simulink model "TBRe18_ECU_V6"  (R2015b)
settings: Solver=FixedStepDiscrete  SolverMode=SingleTasking  StartTime=0.0  StopTime=inf  FixedStep=0.0001  RelTol=1e-3
PostLoadFcn:
  | model_init();
libraries: simulink x20, simulink_extras x1
(part 2 of 4)

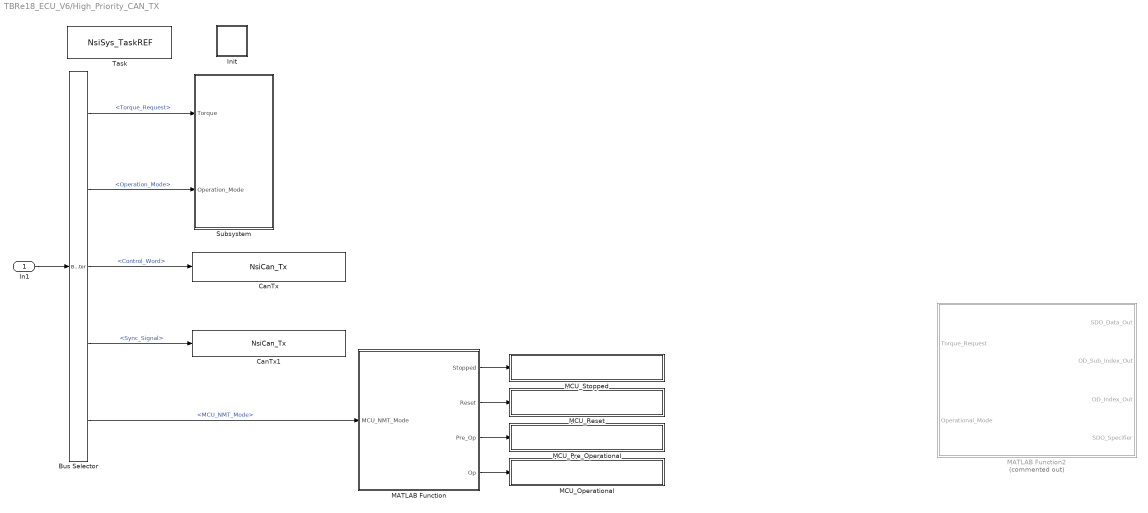
== system TBRe18_ECU_V6/High_Priority_CAN_TX ==
  In1 : Inport
  Bus Selector : BusSelector  OutputSignals=Drive_Data.Torque_Request,Vehicle_Operation_Data.Operation_Mode,Drive_Data.Control_Word,Drive_Data.Sync_Signal,Vehicle_Operation_Data.MCU_NMT_Mode
  CanTx : S-Function  FunctionName=NsiCan_Tx  Parameters=data_can,channel,msg_name,ident,ident_type,dlc,signals  SFunctionDeploymentMode=off  EnableBusSupport=off  mask(MUXlink Can Tx){data_can=1;HIGH_SPEED;500Kbps;120 Ohm;C:\Users\William\Documents\ECU\DBC\TBRe18_DBC_V1.dbc;0;1;HIGH_SPEED;500Kbps;120 Ohm;C:\Users\William\Documents\ECU\DBC\TBRe18_DBC_V1.dbc;0;0;HIGH_SPEED;500Kbps;120 Ohm;C:\Users\l\Desktop\FYP\ECU\DBC\TBRe_DBC_V2.dbc;0;0;HIGH_SPEED;500Kbps;120 Ohm;D:\TOOLS\MUXLINK\R2011b\MUXlink\misc\j1939_adapt.dbc;0;0;HIGH_SPEED;1000Kbps;No;D:\TOOLS\MUXLINK\R2011b\MUXlink\misc\BASE_CAN_MUXLAB4.dbc;0, channel=1, msg_name=MCU_RPDO1, ident=0x201, ident_type=STD, dlc=8, signals=MCU_ControlWord;1;0;16}
      mask prompts: data_can "data can"; msg_name "msg name"
      mask help: Transmit a frame on a CAN Channel.
      mask init:
      | NsiCan_Tx_InitializationFcn();
      settings: OpenFcn=NsiCan_Tx_OpenFcn();
      mask Help:
      | eval('block=get_param(gcb, ''RTWdata'');')
      | web([docroot '\toolbox\MUXlink\html\blocks/' block.MUXlink_BlockType '.html'])
      mask Callback data_can: NsiCan_Tx_ApplyFcn(1);
      mask Callback channel: NsiCan_Tx_ApplyFcn(2);
      mask Callback msg_name: NsiCan_Tx_ApplyFcn(3);
      mask Callback ident: NsiCan_Tx_ApplyFcn(4);
      mask Callback ident_type: NsiCan_Tx_ApplyFcn(5);
      mask Callback dlc: NsiCan_Tx_ApplyFcn(6);
      mask Callback signals: NsiCan_Tx_ApplyFcn(7);
      mask Display: image(imread('nsi.bmp'));text(0.5, 0.1, 'TX_MCU_RPDO1_CAN1', 'horizontalAlignment', 'center', 'verticalAlignment', 'base');plot([0.05 0.05 0.05 0.05 0.05 0.05 0.05 0.05 0.05 0.05]); port_label('input',1, 'MCU_ControlWord');
  CanTx1 : S-Function  FunctionName=NsiCan_Tx  Parameters=data_can,channel,msg_name,ident,ident_type,dlc,signals  SFunctionDeploymentMode=off  EnableBusSupport=off  mask(MUXlink Can Tx){data_can=1;HIGH_SPEED;500Kbps;120 Ohm;C:\Users\William\Documents\ECU\DBC\TBRe18_DBC_V1.dbc;0;1;HIGH_SPEED;500Kbps;120 Ohm;C:\Users\William\Documents\ECU\DBC\TBRe18_DBC_V1.dbc;0;0;HIGH_SPEED;500Kbps;120 Ohm;C:\Users\l\Desktop\FYP\ECU\DBC\TBRe_DBC_V2.dbc;0;0;HIGH_SPEED;500Kbps;120 Ohm;D:\TOOLS\MUXLINK\R2011b\MUXlink\misc\j1939_adapt.dbc;0;0;HIGH_SPEED;1000Kbps;No;D:\TOOLS\MUXLINK\R2011b\MUXlink\misc\BASE_CAN_MUXLAB4.dbc;0, channel=1, msg_name=MCU_Sync_MSG, ident=0x080, ident_type=STD, dlc=1, signals=Sync_Command;1;0;8}
      mask prompts: data_can "data can"; msg_name "msg name"
      mask help: Transmit a frame on a CAN Channel.
      mask init:
      | NsiCan_Tx_InitializationFcn();
      settings: OpenFcn=NsiCan_Tx_OpenFcn();
      mask Help:
      | eval('block=get_param(gcb, ''RTWdata'');')
      | web([docroot '\toolbox\MUXlink\html\blocks/' block.MUXlink_BlockType '.html'])
      mask Callback data_can: NsiCan_Tx_ApplyFcn(1);
      mask Callback channel: NsiCan_Tx_ApplyFcn(2);
      mask Callback msg_name: NsiCan_Tx_ApplyFcn(3);
      mask Callback ident: NsiCan_Tx_ApplyFcn(4);
      mask Callback ident_type: NsiCan_Tx_ApplyFcn(5);
      mask Callback dlc: NsiCan_Tx_ApplyFcn(6);
      mask Callback signals: NsiCan_Tx_ApplyFcn(7);
      mask Display: image(imread('nsi.bmp'));text(0.5, 0.1, 'TX_MCU_Sync_MSG_CAN1', 'horizontalAlignment', 'center', 'verticalAlignment', 'base');plot([0.05 0.05 0.05 0.05 0.05 0.05 0.05 0.05 0.05 0.05]); port_label('input',1, 'Sync_Command');
  Init : Subsystem  mask(System Initialize){}
      mask help: Add code to a systems Initialize function
      settings: CopyFcn=cccopyfcn(gcb)  OpenFcn=ccopenfcn('System Initialize Function')
      mask Help: This block contains text fields to insert custom user code sections at the declaration, execution and exit sections of the systems initialize function.  By placing this block inside a subsytem, the custom user code will appear in that subsystems function.
      mask Display: disp('I()')
  MATLAB Function : MATLAB Function  TreatAsAtomicUnit=on
  MATLAB Function2 : MATLAB Function  Commented=on  TreatAsAtomicUnit=on
  MCU_Operational : Subsystem
  MCU_Pre_Operational : Subsystem
  MCU_Reset : Subsystem
  MCU_Stopped : Subsystem
  Subsystem : Subsystem
  Task : S-Function  FunctionName=NsiSys_TaskREF  Parameters=task_initialised,task_periodic, task_sampletime,task_name,task_event,task_offset  SFunctionDeploymentMode=off  EnableBusSupport=off  mask(task definition){task_initialised=on, task_periodic=on, task_sampletime=[0.1], task_offset=0.03, task_name=High_Priority_CAN_TX, task_event=on}
      mask prompts: task_initialised "task initialised"; task_periodic "Is Periodic"; task_sampletime "Task sample time"; task_offset "Task Offset"; task_name "Task name"; task_event "Is event"
      mask help:
      | Permit to provide all parameters associated to a MUXLINK task.
      | Task can be executed periodicaly and/or on event detection.
      | If task is periodic:
      | Task sample time specify the execution period in mS [0.001   6000]
      | Task Offset specify the offset applied to the execution period
      | Task Offset < Task sample time
      mask init:
      | NsiSys_TaskREF_InitializationFcn();
      settings: OpenFcn=NsiSys_Task_OpenFcn();
      mask Callback task_initialised: NsiSys_TaskREF_ApplyFcn(1);
      mask Callback task_periodic: NsiSys_TaskREF_ApplyFcn(2);
      mask Callback task_sampletime: NsiSys_TaskREF_ApplyFcn(3);
      mask Callback task_offset: NsiSys_TaskREF_ApplyFcn(6);
      mask Callback task_name: NsiSys_TaskREF_ApplyFcn(4);
      mask Callback task_event: NsiSys_TaskREF_ApplyFcn(5);
      mask Display: text(0.5, 0.8, 't()', 'horizontalAlignment', 'center', 'verticalAlignment', 'base');text(0.5, 0.2, '/ 100.0ms / 30.0ms /', 'horizontalAlignment', 'center', 'verticalAlignment', 'base');text(0.5, 0.4, 'Event', 'horizontalAlignment', 'center', 'verticalAlignment', 'base');
  wires:
  In1/1 -> Bus Selector/1
  Bus Selector/4 -> CanTx1/1  "<Sync_Signal>"
  MATLAB Function/4(Op) -> MCU_Operational/Trigger
  MATLAB Function/1(Stopped) -> MCU_Stopped/Trigger
  MATLAB Function/3(Pre_Op) -> MCU_Pre_Operational/Trigger
  Bus Selector/5 -> MATLAB Function/1(MCU_NMT_Mode)  "<MCU_NMT_Mode>"
  Bus Selector/3 -> CanTx/1  "<Control_Word>"
  MATLAB Function/2(Reset) -> MCU_Reset/Trigger
  Bus Selector/2 -> Subsystem/2(Operation_Mode)  "<Operation_Mode>"
  Bus Selector/1 -> Subsystem/1(Torque)  "<Torque_Request>"

== system TBRe18_ECU_V6/Low_Priority_CAN_RX ==
  Bus Creator : BusCreator  Inputs=15
  Bus Creator1 : BusCreator  Inputs=11
  Bus Creator2 : BusCreator  Inputs=2
  CanRx : S-Function  FunctionName=NsiCan_Rx  Parameters=data_can,channel,msg_name,ident,ident_type,dlc,signals,is_trigger  SFunctionDeploymentMode=off  EnableBusSupport=off  mask(MUXlink Can Rx){data_can=1;HIGH_SPEED;500Kbps;120 Ohm;C:\Users\William\Documents\ECU\DBC\TBRe18_DBC_V1.dbc;0;;1;HIGH_SPEED;500Kbps;120 Ohm;C:\Users\William\Documents\ECU\DBC\TBRe18_DBC_V1.dbc;0;;0;HIGH_SPEED;500Kbps;120 Ohm;C:\Users\l\Desktop\FYP\ECU\DBC\TBRe_DBC_V2.dbc;0;;0;HIGH_SPEED;500Kbps;120 Ohm;D:\TOOLS\MUXLINK\R2011b\MUXlink\misc\j1939_adapt.dbc;0;;0;HIGH_SPEED;1000Kbps;No;D:\TOOLS\MUXLINK\R2011b\MUXlink\misc\BASE_CAN_MUXLAB4.dbc;0;, channel=2, msg_name=Shutdown_TPDO, ident=0x185, ident_type=STD, dlc=2, signals=High_AIR_Fault;1;13;1;TSMS_Fault;1;12;1;HVD_Fault;1;11;1;Front_Return_Fault;1;10;1;E2_Switch_Fault;1;9;1;E1_Switch_Fault;1;8;1;Latch_Out_Fault;1;7;1;Latch_In_Fault;1;6;1;BSPD_TSI_Fault;1;5;1;BSPD_Fault;1;4;1;IMD_Fault;1;3;1;BMS_Fault;1;2;1;ESTP_Right_Fault;1;1;1;ESTP_Left_Fault;1;0;1, is_trigger=0}
      mask prompts: data_can "data can"; msg_name "msg name"
      mask help: Receive a frame from a CAN channel.
      mask init:
      | NsiCan_Rx_InitializationFcn();
      settings: OpenFcn=NsiCan_Rx_OpenFcn();
      mask Help:
      | eval('block=get_param(gcb, ''RTWdata'');')
      | web([docroot '\toolbox\MUXlink\html\blocks/' block.MUXlink_BlockType '.html'])
      mask Callback data_can: NsiCan_Rx_ApplyFcn(1);
      mask Callback channel: NsiCan_Rx_ApplyFcn(2);
      mask Callback msg_name: NsiCan_Rx_ApplyFcn(3);
      mask Callback ident: NsiCan_Rx_ApplyFcn(4);
      mask Callback ident_type: NsiCan_Rx_ApplyFcn(5);
      mask Callback dlc: NsiCan_Rx_ApplyFcn(6);
      mask Callback signals: NsiCan_Rx_ApplyFcn(7);
      mask Callback is_trigger: NsiCan_Rx_ApplyFcn(8);
      mask Display: image(imread('nsi.bmp'));text(0.5, 0.3, 'RX_Shutdown_TPDO_CAN2', 'horizontalAlignment', 'center', 'verticalAlignment', 'base');plot([0.05 0.05 0.05 0.05 0.05 0.05 0.05 0.05 0.05 0.05]); port_label('output',1, 'High_AIR_Fault'); port_label('output',2, 'TSMS_Fault'); port_label('output',3, 'HVD_Fault'); port_label('output',4, 'Front_Return_Fault'); port_label('output',5, 'E2_Switch_Fault'); port_label('output',6, 'E1_Switch_Fault'); port_label('output',7, 'Latch_Out_Fault'); port_label('output',8, 'Latch_In_Fault'); port_label('output',9, 'BSPD_TSI_Fault'); port_label('output',10, 'BSPD_Fault'); port_label('output',11, 'IMD_Fault'); port_label('output',12, 'BMS_Fault'); port_label('output',13, 'ESTP_Right_Fault'); port_label('output',14, 'ESTP_Left_Fault'); port_label('output',15, 'Status');
  CanRx1 : S-Function  FunctionName=NsiCan_Rx  Parameters=data_can,channel,msg_name,ident,ident_type,dlc,signals,is_trigger  SFunctionDeploymentMode=off  EnableBusSupport=off  mask(MUXlink Can Rx){data_can=1;HIGH_SPEED;500Kbps;120 Ohm;C:\Users\William\Documents\ECU\DBC\TBRe18_DBC_V1.dbc;0;;1;HIGH_SPEED;500Kbps;120 Ohm;C:\Users\William\Documents\ECU\DBC\TBRe18_DBC_V1.dbc;0;;0;HIGH_SPEED;500Kbps;120 Ohm;C:\Users\l\Desktop\FYP\ECU\DBC\TBRe_DBC_V2.dbc;0;;0;HIGH_SPEED;500Kbps;120 Ohm;D:\TOOLS\MUXLINK\R2011b\MUXlink\misc\j1939_adapt.dbc;0;;0;HIGH_SPEED;1000Kbps;No;D:\TOOLS\MUXLINK\R2011b\MUXlink\misc\BASE_CAN_MUXLAB4.dbc;0;, channel=2, msg_name=BMS_Feedback_1, ident=0x050, ident_type=STD, dlc=7, signals=Instant_Pack_Voltage;1;0;16;Pack_SOC;1;16;16;Pack_Current;1;32;16;Acc_Fan_Speed;1;48;8, is_trigger=0}
      mask prompts: data_can "data can"; msg_name "msg name"
      mask help: Receive a frame from a CAN channel.
      mask init:
      | NsiCan_Rx_InitializationFcn();
      settings: OpenFcn=NsiCan_Rx_OpenFcn();
      mask Help:
      | eval('block=get_param(gcb, ''RTWdata'');')
      | web([docroot '\toolbox\MUXlink\html\blocks/' block.MUXlink_BlockType '.html'])
      mask Callback data_can: NsiCan_Rx_ApplyFcn(1);
      mask Callback channel: NsiCan_Rx_ApplyFcn(2);
      mask Callback msg_name: NsiCan_Rx_ApplyFcn(3);
      mask Callback ident: NsiCan_Rx_ApplyFcn(4);
      mask Callback ident_type: NsiCan_Rx_ApplyFcn(5);
      mask Callback dlc: NsiCan_Rx_ApplyFcn(6);
      mask Callback signals: NsiCan_Rx_ApplyFcn(7);
      mask Callback is_trigger: NsiCan_Rx_ApplyFcn(8);
      mask Display: image(imread('nsi.bmp'));text(0.5, 0.3, 'RX_BMS_Feedback_1_CAN2', 'horizontalAlignment', 'center', 'verticalAlignment', 'base');plot([0.05 0.05 0.05 0.05 0.05 0.05 0.05 0.05 0.05 0.05]); port_label('output',1, 'Instant_Pack_Voltage'); port_label('output',2, 'Pack_SOC'); port_label('output',3, 'Pack_Current'); port_label('output',4, 'Acc_Fan_Speed'); port_label('output',5, 'Status');
  CanRx2 : S-Function  FunctionName=NsiCan_Rx  Parameters=data_can,channel,msg_name,ident,ident_type,dlc,signals,is_trigger  SFunctionDeploymentMode=off  EnableBusSupport=off  mask(MUXlink Can Rx){data_can=1;HIGH_SPEED;500Kbps;120 Ohm;C:\Users\William\Documents\ECU\DBC\TBRe18_DBC_V1.dbc;0;;1;HIGH_SPEED;500Kbps;120 Ohm;C:\Users\William\Documents\ECU\DBC\TBRe18_DBC_V1.dbc;0;;0;HIGH_SPEED;500Kbps;120 Ohm;C:\Users\l\Desktop\FYP\ECU\DBC\TBRe_DBC_V2.dbc;0;;0;HIGH_SPEED;500Kbps;120 Ohm;D:\TOOLS\MUXLINK\R2011b\MUXlink\misc\j1939_adapt.dbc;0;;0;HIGH_SPEED;1000Kbps;No;D:\TOOLS\MUXLINK\R2011b\MUXlink\misc\BASE_CAN_MUXLAB4.dbc;0;, channel=2, msg_name=BMS_Feedback_2, ident=0x051, ident_type=STD, dlc=8, signals=Avg_Cell_Voltage;1;32;16;High_Cell_Voltage;1;16;16;High_Cell_ID;1;56;8;Low_Cell_Voltage;1;0;16;Low_Cell_ID;1;48;8, is_trigger=0}
      mask prompts: data_can "data can"; msg_name "msg name"
      mask help: Receive a frame from a CAN channel.
      mask init:
      | NsiCan_Rx_InitializationFcn();
      settings: OpenFcn=NsiCan_Rx_OpenFcn();
      mask Help:
      | eval('block=get_param(gcb, ''RTWdata'');')
      | web([docroot '\toolbox\MUXlink\html\blocks/' block.MUXlink_BlockType '.html'])
      mask Callback data_can: NsiCan_Rx_ApplyFcn(1);
      mask Callback channel: NsiCan_Rx_ApplyFcn(2);
      mask Callback msg_name: NsiCan_Rx_ApplyFcn(3);
      mask Callback ident: NsiCan_Rx_ApplyFcn(4);
      mask Callback ident_type: NsiCan_Rx_ApplyFcn(5);
      mask Callback dlc: NsiCan_Rx_ApplyFcn(6);
      mask Callback signals: NsiCan_Rx_ApplyFcn(7);
      mask Callback is_trigger: NsiCan_Rx_ApplyFcn(8);
      mask Display: image(imread('nsi.bmp'));text(0.5, 0.3, 'RX_BMS_Feedback_2_CAN2', 'horizontalAlignment', 'center', 'verticalAlignment', 'base');plot([0.05 0.05 0.05 0.05 0.05 0.05 0.05 0.05 0.05 0.05]); port_label('output',1, 'Avg_Cell_Voltage'); port_label('output',2, 'High_Cell_Voltage'); port_label('output',3, 'High_Cell_ID'); port_label('output',4, 'Low_Cell_Voltage'); port_label('output',5, 'Low_Cell_ID'); port_label('output',6, 'Status');
  Init : Subsystem  mask(System Initialize){}
      mask help: Add code to a systems Initialize function
      settings: CopyFcn=cccopyfcn(gcb)  OpenFcn=ccopenfcn('System Initialize Function')
      mask Help: This block contains text fields to insert custom user code sections at the declaration, execution and exit sections of the systems initialize function.  By placing this block inside a subsytem, the custom user code will appear in that subsystems function.
      mask Display: disp('I()')
  Task : S-Function  FunctionName=NsiSys_TaskREF  Parameters=task_initialised,task_periodic, task_sampletime,task_name,task_event,task_offset  SFunctionDeploymentMode=off  EnableBusSupport=off  mask(task definition){task_initialised=on, task_periodic=on, task_sampletime=[0.1], task_offset=0.05, task_name=Low_Priority_CAN_RX, task_event=on}
      mask prompts: task_initialised "task initialised"; task_periodic "Is Periodic"; task_sampletime "Task sample time"; task_offset "Task Offset"; task_name "Task name"; task_event "Is event"
      mask help:
      | Permit to provide all parameters associated to a MUXLINK task.
      | Task can be executed periodicaly and/or on event detection.
      | If task is periodic:
      | Task sample time specify the execution period in mS [0.001   6000]
      | Task Offset specify the offset applied to the execution period
      | Task Offset < Task sample time
      mask init:
      | NsiSys_TaskREF_InitializationFcn();
      settings: OpenFcn=NsiSys_Task_OpenFcn();
      mask Callback task_initialised: NsiSys_TaskREF_ApplyFcn(1);
      mask Callback task_periodic: NsiSys_TaskREF_ApplyFcn(2);
      mask Callback task_sampletime: NsiSys_TaskREF_ApplyFcn(3);
      mask Callback task_offset: NsiSys_TaskREF_ApplyFcn(6);
      mask Callback task_name: NsiSys_TaskREF_ApplyFcn(4);
      mask Callback task_event: NsiSys_TaskREF_ApplyFcn(5);
      mask Display: text(0.5, 0.8, 't()', 'horizontalAlignment', 'center', 'verticalAlignment', 'base');text(0.5, 0.2, '/ 100.0ms / 50.0ms /', 'horizontalAlignment', 'center', 'verticalAlignment', 'base');text(0.5, 0.4, 'Event', 'horizontalAlignment', 'center', 'verticalAlignment', 'base');
  UsbTx : S-Function  FunctionName=NsiUsb_Tx  Parameters=signame,resolution,offset,unite  SFunctionDeploymentMode=off  EnableBusSupport=off  mask(MUXlink Usb Tx){signame=Speed, resolution=1, offset=0, unite=km/h}
      mask prompts: signame "Signal name ?"; resolution "Resolution ?"; offset "Offset ?"; unite "Unit ?"
      mask help: Transmit a frame on the USB Channel.
      mask init:
      | NsiUsb_Tx_InitializationFcn();
      settings: OpenFcn=NsiUsb_Tx_OpenFcn();
      mask Help:
      | eval('block=get_param(gcb, ''RTWdata'');')
      | web([docroot '\toolbox\MUXlink\html\blocks/' block.MUXlink_BlockType '.html'])
      mask Callback signame: NsiUsb_Tx_ApplyFcn(1);
      mask Callback resolution: NsiUsb_Tx_ApplyFcn(2);
      mask Callback offset: NsiUsb_Tx_ApplyFcn(3);
      mask Callback unite: NsiUsb_Tx_ApplyFcn(4);
      mask Display: image(imread('nsi.bmp'));text(0.5, 0.2, 'USB Tx', 'horizontalAlignment', 'center', 'verticalAlignment', 'base');plot([0.05 0.05 0.05 0.05 0.05 0.05 0.05 0.05 0.05 0.05]);port_label('input',1, 'Speed');
  Out1 : Outport
  wires:
  CanRx/15 -> Bus Creator/15  "Shutdown_Status"
  CanRx/14 -> Bus Creator/14  "ESTP_Left_Fault"
  CanRx/12 -> Bus Creator/12  "BMS_Fault"
  CanRx/13 -> Bus Creator/13  "ESTP_Right_Fault"
  CanRx/1 -> Bus Creator/1  "High_AIR_Fault"
  CanRx/2 -> Bus Creator/2  "TSMS_Fault"
  CanRx/3 -> Bus Creator/3  "HVD_Fault"
  CanRx/4 -> Bus Creator/4  "Front_Return_Fault"
  CanRx/5 -> Bus Creator/5  "E2_Switch_Fault"
  CanRx/6 -> Bus Creator/6  "E1_Switch_Fault"
  CanRx/7 -> Bus Creator/7  "Latch_Out_Fault"
  CanRx/8 -> Bus Creator/8  "Latch_In_Fault"
  CanRx/9 -> Bus Creator/9  "BSPD_TSI_Fault"
  CanRx/10 -> Bus Creator/10  "BSPD_Fault"
  CanRx/11 -> Bus Creator/11  "IMD_Fault"
  Bus Creator/1 -> Bus Creator2/1  "Shutdown_Data"
  Bus Creator2/1 -> Out1/1
  CanRx1/1 -> Bus Creator1/1  "Instant_Pack_Voltage"
  CanRx1/2 -> Bus Creator1/2  "Pack_SOC"
  CanRx1/3 -> Bus Creator1/3  "Pack_Current"
  CanRx1/4 -> Bus Creator1/4  "Acc_Fan_Speed"
  CanRx2/1 -> Bus Creator1/6  "Abg_Cell_Voltage"
  CanRx2/2 -> Bus Creator1/7  "High_Cell_Voltage"
  CanRx2/3 -> Bus Creator1/8  "High_Cell_ID"
  CanRx2/4 -> Bus Creator1/9  "Low_Cell_Voltage"
  CanRx2/5 -> UsbTx/1, Bus Creator1/10  "Low_Cell_ID"
  CanRx1/5 -> Bus Creator1/5
  CanRx2/6 -> Bus Creator1/11
  Bus Creator1/1 -> Bus Creator2/2  "BMS_Data"

== system TBRe18_ECU_V6/Low_Priority_CAN_TX ==
  In1 : Inport
  BMS_Diagnostics_Data : Subsystem
  CSB_Data : Subsystem
  ECU_Data : Subsystem
  Init : Subsystem  mask(System Initialize){}
      mask help: Add code to a systems Initialize function
      settings: CopyFcn=cccopyfcn(gcb)  OpenFcn=ccopenfcn('System Initialize Function')
      mask Help: This block contains text fields to insert custom user code sections at the declaration, execution and exit sections of the systems initialize function.  By placing this block inside a subsytem, the custom user code will appear in that subsystems function.
      mask Display: disp('I()')
  MCU_Data : Subsystem
  Shutdown_System_Data : Subsystem
  Task : S-Function  FunctionName=NsiSys_TaskREF  Parameters=task_initialised,task_periodic, task_sampletime,task_name,task_event,task_offset  SFunctionDeploymentMode=off  EnableBusSupport=off  mask(task definition){task_initialised=on, task_periodic=on, task_sampletime=[0.1], task_offset=0.03, task_name=Low_Priority_CAN_TX, task_event=on}
      mask prompts: task_initialised "task initialised"; task_periodic "Is Periodic"; task_sampletime "Task sample time"; task_offset "Task Offset"; task_name "Task name"; task_event "Is event"
      mask help:
      | Permit to provide all parameters associated to a MUXLINK task.
      | Task can be executed periodicaly and/or on event detection.
      | If task is periodic:
      | Task sample time specify the execution period in mS [0.001   6000]
      | Task Offset specify the offset applied to the execution period
      | Task Offset < Task sample time
      mask init:
      | NsiSys_TaskREF_InitializationFcn();
      settings: OpenFcn=NsiSys_Task_OpenFcn();
      mask Callback task_initialised: NsiSys_TaskREF_ApplyFcn(1);
      mask Callback task_periodic: NsiSys_TaskREF_ApplyFcn(2);
      mask Callback task_sampletime: NsiSys_TaskREF_ApplyFcn(3);
      mask Callback task_offset: NsiSys_TaskREF_ApplyFcn(6);
      mask Callback task_name: NsiSys_TaskREF_ApplyFcn(4);
      mask Callback task_event: NsiSys_TaskREF_ApplyFcn(5);
      mask Display: text(0.5, 0.8, 't()', 'horizontalAlignment', 'center', 'verticalAlignment', 'base');text(0.5, 0.2, '/ 100.0ms / 30.0ms /', 'horizontalAlignment', 'center', 'verticalAlignment', 'base');text(0.5, 0.4, 'Event', 'horizontalAlignment', 'center', 'verticalAlignment', 'base');
  wires:
  In1/1 -> CSB_Data/1(In1), BMS_Diagnostics_Data/1(In1), Shutdown_System_Data/1(In1), ECU_Data/1(In1), MCU_Data/1(In1)

== system TBRe18_ECU_V6/Data_Processing/Diagnostics ==
  note: Diagnostics
  Raw_Input_Data : Inport
  BMS_Diagnostics : Subsystem
  Bus Creator : BusCreator  Inputs=5
  ECU_I/0s_Diagnostics : Subsystem
  MCU_Diagnostics : Subsystem
  Shutdown_System_Diagnostics : Subsystem
  Input_Data_Bus : Outport
  wires:
  Bus Creator/1 -> Input_Data_Bus/1
  Raw_Input_Data/1 -> BMS_Diagnostics/1(In1), Shutdown_System_Diagnostics/1(In1), ECU_I/0s_Diagnostics/1(In1), MCU_Diagnostics/1(In1), Bus Creator/1  "Raw_Input_Data"
  BMS_Diagnostics/1(Out1) -> Bus Creator/5  "BMS_Data"
  Shutdown_System_Diagnostics/1(Out1) -> Bus Creator/4  "Shutdown_Data"
  ECU_I/0s_Diagnostics/1(Out1) -> Bus Creator/3  "ECU_IO_Data"
  MCU_Diagnostics/1(Out1) -> Bus Creator/2  "MCU_Data"

== system TBRe18_ECU_V6/Data_Processing/Init ==

== system TBRe18_ECU_V6/Data_Processing/Vehicle_Functionality ==
  note: Vehicle_Functionality
  Input_Data : Inport
  Bus Creator : BusCreator  Inputs=4
  Drive_Function : Subsystem
  Hardwired_Output_Functions : Subsystem
  Vehicle_Operation_Mode : Subsystem
  Output_Data_Bus : Outport
  wires:
  Input_Data/1 -> Hardwired_Output_Functions/1(In1), Drive_Function/1(Data_In), Vehicle_Operation_Mode/1(Diagnostic_Data), Bus Creator/1  "Input_Data_Bus"
  Vehicle_Operation_Mode/1(Data_Out) -> Hardwired_Output_Functions/2(Vehicle_Operation_Data), Drive_Function/2(Vehicle_Operation_Data), Bus Creator/2  "Vehicle_Operation_Data"
  Hardwired_Output_Functions/1(Out1) -> Bus Creator/4  "Hardwired_Output_Data"
  Drive_Function/1(Drive_Data) -> Bus Creator/3  "Drive_Data"
  Bus Creator/1 -> Output_Data_Bus/1

== system TBRe18_ECU_V6/Hardwired_Inputs/Console ==
  Bus Creator : BusCreator  Inputs=2
  DigitalInput : S-Function  FunctionName=NsiIo_DigitalInput  Parameters=channel,is_trigger,typeof_trigger,is_wakeup,wakeup_level  SFunctionDeploymentMode=off  EnableBusSupport=off  mask(MUXlink I/O Digital Input){channel=3, is_trigger=off, typeof_trigger=Either, is_wakeup=off, wakeup_level=Low level}
      mask prompts: channel "Channel ?"; is_trigger "Trigger ?"; typeof_trigger "Type of Trigger ?"; is_wakeup "Wake-up ?"; wakeup_level "Wake-up level ?"
      mask help: Read digital input from I/O channel.
      mask init:
      | NsiIo_DigitalInput_InitializationFcn();
      settings: OpenFcn=NsiIo_DigitalInput_OpenFcn();
      mask Help:
      | eval('block=get_param(gcb, ''RTWdata'');')
      | web([docroot '\toolbox\MUXlink\html\blocks/' block.MUXlink_BlockType '.html'])
      mask Callback channel: NsiIo_DigitalInput_ApplyFcn(1);
      mask Callback is_trigger: NsiIo_DigitalInput_ApplyFcn(2);
      mask TypeOptions typeof_trigger: Rising | Falling | Either
      mask Callback typeof_trigger: NsiIo_DigitalInput_ApplyFcn(3);
      mask Callback is_wakeup: NsiIo_DigitalInput_ApplyFcn(4);
      mask TypeOptions wakeup_level: Low level | High level
      mask Callback wakeup_level: NsiIo_DigitalInput_ApplyFcn(5);
      mask Display: image(imread('nsi.bmp'));text(0.5, 0.2, 'DigitalInput_3', 'horizontalAlignment', 'center', 'verticalAlignment', 'base');plot([0.05 0.05 0.05 0.05 0.05 0.05 0.05 0.05 0.05 0.05]);port_label('output', 1, 'Ground : A3');
  DigitalInput1 : S-Function  FunctionName=NsiIo_DigitalInput  Parameters=channel,is_trigger,typeof_trigger,is_wakeup,wakeup_level  SFunctionDeploymentMode=off  EnableBusSupport=off  mask(MUXlink I/O Digital Input){channel=2, is_trigger=off, typeof_trigger=Either, is_wakeup=off, wakeup_level=Low level}
      mask prompts: channel "Channel ?"; is_trigger "Trigger ?"; typeof_trigger "Type of Trigger ?"; is_wakeup "Wake-up ?"; wakeup_level "Wake-up level ?"
      mask help: Read digital input from I/O channel.
      mask init:
      | NsiIo_DigitalInput_InitializationFcn();
      settings: OpenFcn=NsiIo_DigitalInput_OpenFcn();
      mask Help:
      | eval('block=get_param(gcb, ''RTWdata'');')
      | web([docroot '\toolbox\MUXlink\html\blocks/' block.MUXlink_BlockType '.html'])
      mask Callback channel: NsiIo_DigitalInput_ApplyFcn(1);
      mask Callback is_trigger: NsiIo_DigitalInput_ApplyFcn(2);
      mask TypeOptions typeof_trigger: Rising | Falling | Either
      mask Callback typeof_trigger: NsiIo_DigitalInput_ApplyFcn(3);
      mask Callback is_wakeup: NsiIo_DigitalInput_ApplyFcn(4);
      mask TypeOptions wakeup_level: Low level | High level
      mask Callback wakeup_level: NsiIo_DigitalInput_ApplyFcn(5);
      mask Display: image(imread('nsi.bmp'));text(0.5, 0.2, 'DigitalInput_2', 'horizontalAlignment', 'center', 'verticalAlignment', 'base');plot([0.05 0.05 0.05 0.05 0.05 0.05 0.05 0.05 0.05 0.05]);port_label('output', 1, 'Ground : A2');
  Out1 : Outport
  wires:
  Bus Creator/1 -> Out1/1
  DigitalInput1/1 -> Bus Creator/2  "Push_to_Start"
  DigitalInput/1 -> Bus Creator/1  "Reset"

== system TBRe18_ECU_V6/Hardwired_Inputs/Init ==

== system TBRe18_ECU_V6/Hardwired_Inputs/Pedal_Box ==
  AnalogInput : S-Function  FunctionName=NsiIo_AnalogInput  Parameters=channel  SFunctionDeploymentMode=off  EnableBusSupport=off  mask(MUXlink I/O Analog Input){channel=1}
      mask prompts: channel "Channel ?"
      mask help: Read analogic input from ADC channel.
      mask init:
      | NsiIo_AnalogInput_InitializationFcn();
      settings: OpenFcn=NsiIo_AnalogInput_OpenFcn();
      mask Help:
      | eval('block=get_param(gcb, ''RTWdata'');')
      | web([docroot '\toolbox\MUXlink\html\blocks/' block.MUXlink_BlockType '.html'])
      mask Callback channel: NsiIo_AnalogInput_ApplyFcn(1);
      mask Display: image(imread('nsi.bmp'));text(0.5, 0.2, 'AnalogInput_1', 'horizontalAlignment', 'center', 'verticalAlignment', 'base');plot([0.05 0.05 0.05 0.05 0.05 0.05 0.05 0.05 0.05 0.05]);port_label('output', 1, 'B1');
  AnalogInput1 : S-Function  FunctionName=NsiIo_AnalogInput  Parameters=channel  SFunctionDeploymentMode=off  EnableBusSupport=off  mask(MUXlink I/O Analog Input){channel=3}
      mask prompts: channel "Channel ?"
      mask help: Read analogic input from ADC channel.
      mask init:
      | NsiIo_AnalogInput_InitializationFcn();
      settings: OpenFcn=NsiIo_AnalogInput_OpenFcn();
      mask Help:
      | eval('block=get_param(gcb, ''RTWdata'');')
      | web([docroot '\toolbox\MUXlink\html\blocks/' block.MUXlink_BlockType '.html'])
      mask Callback channel: NsiIo_AnalogInput_ApplyFcn(1);
      mask Display: image(imread('nsi.bmp'));text(0.5, 0.2, 'AnalogInput_3', 'horizontalAlignment', 'center', 'verticalAlignment', 'base');plot([0.05 0.05 0.05 0.05 0.05 0.05 0.05 0.05 0.05 0.05]);port_label('output', 1, 'B3');
  AnalogInput2 : S-Function  FunctionName=NsiIo_AnalogInput  Parameters=channel  SFunctionDeploymentMode=off  EnableBusSupport=off  mask(MUXlink I/O Analog Input){channel=2}
      mask prompts: channel "Channel ?"
      mask help: Read analogic input from ADC channel.
      mask init:
      | NsiIo_AnalogInput_InitializationFcn();
      settings: OpenFcn=NsiIo_AnalogInput_OpenFcn();
      mask Help:
      | eval('block=get_param(gcb, ''RTWdata'');')
      | web([docroot '\toolbox\MUXlink\html\blocks/' block.MUXlink_BlockType '.html'])
      mask Callback channel: NsiIo_AnalogInput_ApplyFcn(1);
      mask Display: image(imread('nsi.bmp'));text(0.5, 0.2, 'AnalogInput_2', 'horizontalAlignment', 'center', 'verticalAlignment', 'base');plot([0.05 0.05 0.05 0.05 0.05 0.05 0.05 0.05 0.05 0.05]);port_label('output', 1, 'B2');
  AnalogInput3 : S-Function  FunctionName=NsiIo_AnalogInput  Parameters=channel  SFunctionDeploymentMode=off  EnableBusSupport=off  mask(MUXlink I/O Analog Input){channel=5}
      mask prompts: channel "Channel ?"
      mask help: Read analogic input from ADC channel.
      mask init:
      | NsiIo_AnalogInput_InitializationFcn();
      settings: OpenFcn=NsiIo_AnalogInput_OpenFcn();
      mask Help:
      | eval('block=get_param(gcb, ''RTWdata'');')
      | web([docroot '\toolbox\MUXlink\html\blocks/' block.MUXlink_BlockType '.html'])
      mask Callback channel: NsiIo_AnalogInput_ApplyFcn(1);
      mask Display: image(imread('nsi.bmp'));text(0.5, 0.2, 'AnalogInput_5', 'horizontalAlignment', 'center', 'verticalAlignment', 'base');plot([0.05 0.05 0.05 0.05 0.05 0.05 0.05 0.05 0.05 0.05]);port_label('output', 1, 'C3');
  AnalogInput4 : S-Function  FunctionName=NsiIo_AnalogInput  Parameters=channel  SFunctionDeploymentMode=off  EnableBusSupport=off  mask(MUXlink I/O Analog Input){channel=6}
      mask prompts: channel "Channel ?"
      mask help: Read analogic input from ADC channel.
      mask init:
      | NsiIo_AnalogInput_InitializationFcn();
      settings: OpenFcn=NsiIo_AnalogInput_OpenFcn();
      mask Help:
      | eval('block=get_param(gcb, ''RTWdata'');')
      | web([docroot '\toolbox\MUXlink\html\blocks/' block.MUXlink_BlockType '.html'])
      mask Callback channel: NsiIo_AnalogInput_ApplyFcn(1);
      mask Display: image(imread('nsi.bmp'));text(0.5, 0.2, 'AnalogInput_6', 'horizontalAlignment', 'center', 'verticalAlignment', 'base');plot([0.05 0.05 0.05 0.05 0.05 0.05 0.05 0.05 0.05 0.05]);port_label('output', 1, 'C4');
  Bus Creator : BusCreator  Inputs=5
  UsbTx : S-Function  FunctionName=NsiUsb_Tx  Parameters=signame,resolution,offset,unite  SFunctionDeploymentMode=off  EnableBusSupport=off  mask(MUXlink Usb Tx){signame=Throttle 1, resolution=1, offset=0, unite=mV}
      mask prompts: signame "Signal name ?"; resolution "Resolution ?"; offset "Offset ?"; unite "Unit ?"
      mask help: Transmit a frame on the USB Channel.
      mask init:
      | NsiUsb_Tx_InitializationFcn();
      settings: OpenFcn=NsiUsb_Tx_OpenFcn();
      mask Help:
      | eval('block=get_param(gcb, ''RTWdata'');')
      | web([docroot '\toolbox\MUXlink\html\blocks/' block.MUXlink_BlockType '.html'])
      mask Callback signame: NsiUsb_Tx_ApplyFcn(1);
      mask Callback resolution: NsiUsb_Tx_ApplyFcn(2);
      mask Callback offset: NsiUsb_Tx_ApplyFcn(3);
      mask Callback unite: NsiUsb_Tx_ApplyFcn(4);
      mask Display: image(imread('nsi.bmp'));text(0.5, 0.2, 'USB Tx', 'horizontalAlignment', 'center', 'verticalAlignment', 'base');plot([0.05 0.05 0.05 0.05 0.05 0.05 0.05 0.05 0.05 0.05]);port_label('input',1, 'Throttle 1');
  UsbTx1 : S-Function  FunctionName=NsiUsb_Tx  Parameters=signame,resolution,offset,unite  SFunctionDeploymentMode=off  EnableBusSupport=off  mask(MUXlink Usb Tx){signame=Throttle 2, resolution=1, offset=0, unite=mV}
      mask prompts: signame "Signal name ?"; resolution "Resolution ?"; offset "Offset ?"; unite "Unit ?"
      mask help: Transmit a frame on the USB Channel.
      mask init:
      | NsiUsb_Tx_InitializationFcn();
      settings: OpenFcn=NsiUsb_Tx_OpenFcn();
      mask Help:
      | eval('block=get_param(gcb, ''RTWdata'');')
      | web([docroot '\toolbox\MUXlink\html\blocks/' block.MUXlink_BlockType '.html'])
      mask Callback signame: NsiUsb_Tx_ApplyFcn(1);
      mask Callback resolution: NsiUsb_Tx_ApplyFcn(2);
      mask Callback offset: NsiUsb_Tx_ApplyFcn(3);
      mask Callback unite: NsiUsb_Tx_ApplyFcn(4);
      mask Display: image(imread('nsi.bmp'));text(0.5, 0.2, 'USB Tx', 'horizontalAlignment', 'center', 'verticalAlignment', 'base');plot([0.05 0.05 0.05 0.05 0.05 0.05 0.05 0.05 0.05 0.05]);port_label('input',1, 'Throttle 2');
  UsbTx2 : S-Function  FunctionName=NsiUsb_Tx  Parameters=signame,resolution,offset,unite  SFunctionDeploymentMode=off  EnableBusSupport=off  mask(MUXlink Usb Tx){signame=Brake, resolution=1, offset=0, unite=mV}
      mask prompts: signame "Signal name ?"; resolution "Resolution ?"; offset "Offset ?"; unite "Unit ?"
      mask help: Transmit a frame on the USB Channel.
      mask init:
      | NsiUsb_Tx_InitializationFcn();
      settings: OpenFcn=NsiUsb_Tx_OpenFcn();
      mask Help:
      | eval('block=get_param(gcb, ''RTWdata'');')
      | web([docroot '\toolbox\MUXlink\html\blocks/' block.MUXlink_BlockType '.html'])
      mask Callback signame: NsiUsb_Tx_ApplyFcn(1);
      mask Callback resolution: NsiUsb_Tx_ApplyFcn(2);
      mask Callback offset: NsiUsb_Tx_ApplyFcn(3);
      mask Callback unite: NsiUsb_Tx_ApplyFcn(4);
      mask Display: image(imread('nsi.bmp'));text(0.5, 0.2, 'USB Tx', 'horizontalAlignment', 'center', 'verticalAlignment', 'base');plot([0.05 0.05 0.05 0.05 0.05 0.05 0.05 0.05 0.05 0.05]);port_label('input',1, 'Brake');
  Out1 : Outport
  wires:
  AnalogInput2/1 -> UsbTx1/1, Bus Creator/2  "Throttle2_Voltage"
  AnalogInput/1 -> UsbTx/1, Bus Creator/1  "Throttle1_Voltage"
  AnalogInput1/1 -> UsbTx2/1, Bus Creator/3  "Brake_Voltage"
  Bus Creator/1 -> Out1/1
  AnalogInput3/1 -> Bus Creator/4  "BSPD_Brake"
  AnalogInput4/1 -> Bus Creator/5  "BSPD_Current"

== system TBRe18_ECU_V6/Hardwired_Outputs/Init ==

== system TBRe18_ECU_V6/High_Priority_CAN_RX/Init ==

== system TBRe18_ECU_V6/High_Priority_CAN_TX/Init ==

== system TBRe18_ECU_V6/High_Priority_CAN_TX/MCU_Operational ==
  Trigger : TriggerPort  PortDimensions=1
  0_constant : Constant  Value=0  OutDataTypeStr=uint8  SampleTime=-1
  0_constant1 : Constant  OutDataTypeStr=uint8  SampleTime=-1
  CanTx : S-Function  FunctionName=NsiCan_Tx  Parameters=data_can,channel,msg_name,ident,ident_type,dlc,signals  SFunctionDeploymentMode=off  EnableBusSupport=off  mask(MUXlink Can Tx){data_can=1;HIGH_SPEED;500Kbps;120 Ohm;C:\Users\William\Documents\ECU\DBC\TBRe18_DBC_V1.dbc;0;0;HIGH_SPEED;500Kbps;120 Ohm;C:\Users\William\Documents\ECU\DBC\TBRe18_DBC_V1.dbc;0;0;HIGH_SPEED;500Kbps;120 Ohm;C:\Users\l\Desktop\FYP\ECU\DBC\TBRe_DBC_V2.dbc;0;0;HIGH_SPEED;500Kbps;120 Ohm;D:\TOOLS\MUXLINK\R2011b\MUXlink\misc\j1939_adapt.dbc;0;0;HIGH_SPEED;1000Kbps;No;D:\TOOLS\MUXLINK\R2011b\MUXlink\misc\BASE_CAN_MUXLAB4.dbc;0, channel=1, msg_name=NMT_Broadcast, ident=0x000, ident_type=STD, dlc=2, signals=NMT_Command;1;0;8;NMT_Command_0;1;8;8}
      mask prompts: data_can "data can"; msg_name "msg name"
      mask help: Transmit a frame on a CAN Channel.
      mask init:
      | NsiCan_Tx_InitializationFcn();
      settings: OpenFcn=NsiCan_Tx_OpenFcn();
      mask Help:
      | eval('block=get_param(gcb, ''RTWdata'');')
      | web([docroot '\toolbox\MUXlink\html\blocks/' block.MUXlink_BlockType '.html'])
      mask Callback data_can: NsiCan_Tx_ApplyFcn(1);
      mask Callback channel: NsiCan_Tx_ApplyFcn(2);
      mask Callback msg_name: NsiCan_Tx_ApplyFcn(3);
      mask Callback ident: NsiCan_Tx_ApplyFcn(4);
      mask Callback ident_type: NsiCan_Tx_ApplyFcn(5);
      mask Callback dlc: NsiCan_Tx_ApplyFcn(6);
      mask Callback signals: NsiCan_Tx_ApplyFcn(7);
      mask Display: image(imread('nsi.bmp'));text(0.5, 0.3, 'TX_NMT_Broadcast_CAN1', 'horizontalAlignment', 'center', 'verticalAlignment', 'base');plot([0.05 0.05 0.05 0.05 0.05 0.05 0.05 0.05 0.05 0.05]); port_label('input',1, 'NMT_Command'); port_label('input',2, 'NMT_Command_0');
  wires:
  0_constant/1 -> CanTx/2
  0_constant1/1 -> CanTx/1

== system TBRe18_ECU_V6/High_Priority_CAN_TX/MCU_Pre_Operational ==
  Trigger : TriggerPort  PortDimensions=1
  0_constant : Constant  Value=0  OutDataTypeStr=uint8  SampleTime=-1
  0_constant1 : Constant  Value=128  OutDataTypeStr=uint8  SampleTime=-1
  CanTx : S-Function  FunctionName=NsiCan_Tx  Parameters=data_can,channel,msg_name,ident,ident_type,dlc,signals  SFunctionDeploymentMode=off  EnableBusSupport=off  mask(MUXlink Can Tx){data_can=1;HIGH_SPEED;500Kbps;120 Ohm;C:\Users\William\Documents\ECU\DBC\TBRe18_DBC_V1.dbc;0;0;HIGH_SPEED;500Kbps;120 Ohm;C:\Users\William\Documents\ECU\DBC\TBRe18_DBC_V1.dbc;0;0;HIGH_SPEED;500Kbps;120 Ohm;C:\Users\l\Desktop\FYP\ECU\DBC\TBRe_DBC_V2.dbc;0;0;HIGH_SPEED;500Kbps;120 Ohm;D:\TOOLS\MUXLINK\R2011b\MUXlink\misc\j1939_adapt.dbc;0;0;HIGH_SPEED;1000Kbps;No;D:\TOOLS\MUXLINK\R2011b\MUXlink\misc\BASE_CAN_MUXLAB4.dbc;0, channel=1, msg_name=NMT_Broadcast, ident=0x000, ident_type=STD, dlc=2, signals=NMT_Command;1;0;8;NMT_Command_0;1;8;8}
      mask prompts: data_can "data can"; msg_name "msg name"
      mask help: Transmit a frame on a CAN Channel.
      mask init:
      | NsiCan_Tx_InitializationFcn();
      settings: OpenFcn=NsiCan_Tx_OpenFcn();
      mask Help:
      | eval('block=get_param(gcb, ''RTWdata'');')
      | web([docroot '\toolbox\MUXlink\html\blocks/' block.MUXlink_BlockType '.html'])
      mask Callback data_can: NsiCan_Tx_ApplyFcn(1);
      mask Callback channel: NsiCan_Tx_ApplyFcn(2);
      mask Callback msg_name: NsiCan_Tx_ApplyFcn(3);
      mask Callback ident: NsiCan_Tx_ApplyFcn(4);
      mask Callback ident_type: NsiCan_Tx_ApplyFcn(5);
      mask Callback dlc: NsiCan_Tx_ApplyFcn(6);
      mask Callback signals: NsiCan_Tx_ApplyFcn(7);
      mask Display: image(imread('nsi.bmp'));text(0.5, 0.3, 'TX_NMT_Broadcast_CAN1', 'horizontalAlignment', 'center', 'verticalAlignment', 'base');plot([0.05 0.05 0.05 0.05 0.05 0.05 0.05 0.05 0.05 0.05]); port_label('input',1, 'NMT_Command'); port_label('input',2, 'NMT_Command_0');
  wires:
  0_constant/1 -> CanTx/2
  0_constant1/1 -> CanTx/1

== system TBRe18_ECU_V6/High_Priority_CAN_TX/MCU_Reset ==
  Trigger : TriggerPort  PortDimensions=1
  0_constant : Constant  Value=0  OutDataTypeStr=uint8  SampleTime=-1
  0_constant1 : Constant  Value=129  OutDataTypeStr=uint8  SampleTime=-1
  CanTx : S-Function  FunctionName=NsiCan_Tx  Parameters=data_can,channel,msg_name,ident,ident_type,dlc,signals  SFunctionDeploymentMode=off  EnableBusSupport=off  mask(MUXlink Can Tx){data_can=1;HIGH_SPEED;500Kbps;120 Ohm;C:\Users\William\Documents\ECU\DBC\TBRe18_DBC_V1.dbc;0;0;HIGH_SPEED;500Kbps;120 Ohm;C:\Users\William\Documents\ECU\DBC\TBRe18_DBC_V1.dbc;0;0;HIGH_SPEED;500Kbps;120 Ohm;C:\Users\l\Desktop\FYP\ECU\DBC\TBRe_DBC_V2.dbc;0;0;HIGH_SPEED;500Kbps;120 Ohm;D:\TOOLS\MUXLINK\R2011b\MUXlink\misc\j1939_adapt.dbc;0;0;HIGH_SPEED;1000Kbps;No;D:\TOOLS\MUXLINK\R2011b\MUXlink\misc\BASE_CAN_MUXLAB4.dbc;0, channel=1, msg_name=NMT_Broadcast, ident=0x000, ident_type=STD, dlc=2, signals=NMT_Command;1;0;8;NMT_Command_0;1;8;8}
      mask prompts: data_can "data can"; msg_name "msg name"
      mask help: Transmit a frame on a CAN Channel.
      mask init:
      | NsiCan_Tx_InitializationFcn();
      settings: OpenFcn=NsiCan_Tx_OpenFcn();
      mask Help:
      | eval('block=get_param(gcb, ''RTWdata'');')
      | web([docroot '\toolbox\MUXlink\html\blocks/' block.MUXlink_BlockType '.html'])
      mask Callback data_can: NsiCan_Tx_ApplyFcn(1);
      mask Callback channel: NsiCan_Tx_ApplyFcn(2);
      mask Callback msg_name: NsiCan_Tx_ApplyFcn(3);
      mask Callback ident: NsiCan_Tx_ApplyFcn(4);
      mask Callback ident_type: NsiCan_Tx_ApplyFcn(5);
      mask Callback dlc: NsiCan_Tx_ApplyFcn(6);
      mask Callback signals: NsiCan_Tx_ApplyFcn(7);
      mask Display: image(imread('nsi.bmp'));text(0.5, 0.3, 'TX_NMT_Broadcast_CAN1', 'horizontalAlignment', 'center', 'verticalAlignment', 'base');plot([0.05 0.05 0.05 0.05 0.05 0.05 0.05 0.05 0.05 0.05]); port_label('input',1, 'NMT_Command'); port_label('input',2, 'NMT_Command_0');
  wires:
  0_constant/1 -> CanTx/2
  0_constant1/1 -> CanTx/1

== system TBRe18_ECU_V6/High_Priority_CAN_TX/MCU_Stopped ==
  Trigger : TriggerPort  PortDimensions=1
  0_constant : Constant  Value=0  OutDataTypeStr=uint8  SampleTime=-1
  0_constant1 : Constant  Value=2  OutDataTypeStr=uint8  SampleTime=-1
  CanTx : S-Function  FunctionName=NsiCan_Tx  Parameters=data_can,channel,msg_name,ident,ident_type,dlc,signals  SFunctionDeploymentMode=off  EnableBusSupport=off  mask(MUXlink Can Tx){data_can=1;HIGH_SPEED;500Kbps;120 Ohm;C:\Users\William\Documents\ECU\DBC\TBRe18_DBC_V1.dbc;0;0;HIGH_SPEED;500Kbps;120 Ohm;C:\Users\William\Documents\ECU\DBC\TBRe18_DBC_V1.dbc;0;0;HIGH_SPEED;500Kbps;120 Ohm;C:\Users\l\Desktop\FYP\ECU\DBC\TBRe_DBC_V2.dbc;0;0;HIGH_SPEED;500Kbps;120 Ohm;D:\TOOLS\MUXLINK\R2011b\MUXlink\misc\j1939_adapt.dbc;0;0;HIGH_SPEED;1000Kbps;No;D:\TOOLS\MUXLINK\R2011b\MUXlink\misc\BASE_CAN_MUXLAB4.dbc;0, channel=1, msg_name=NMT_Broadcast, ident=0x000, ident_type=STD, dlc=2, signals=NMT_Command;1;0;8;NMT_Command_0;1;8;8}
      mask prompts: data_can "data can"; msg_name "msg name"
      mask help: Transmit a frame on a CAN Channel.
      mask init:
      | NsiCan_Tx_InitializationFcn();
      settings: OpenFcn=NsiCan_Tx_OpenFcn();
      mask Help:
      | eval('block=get_param(gcb, ''RTWdata'');')
      | web([docroot '\toolbox\MUXlink\html\blocks/' block.MUXlink_BlockType '.html'])
      mask Callback data_can: NsiCan_Tx_ApplyFcn(1);
      mask Callback channel: NsiCan_Tx_ApplyFcn(2);
      mask Callback msg_name: NsiCan_Tx_ApplyFcn(3);
      mask Callback ident: NsiCan_Tx_ApplyFcn(4);
      mask Callback ident_type: NsiCan_Tx_ApplyFcn(5);
      mask Callback dlc: NsiCan_Tx_ApplyFcn(6);
      mask Callback signals: NsiCan_Tx_ApplyFcn(7);
      mask Display: image(imread('nsi.bmp'));text(0.5, 0.3, 'TX_NMT_Broadcast_CAN1', 'horizontalAlignment', 'center', 'verticalAlignment', 'base');plot([0.05 0.05 0.05 0.05 0.05 0.05 0.05 0.05 0.05 0.05]); port_label('input',1, 'NMT_Command'); port_label('input',2, 'NMT_Command_0');
  wires:
  0_constant/1 -> CanTx/2
  0_constant1/1 -> CanTx/1

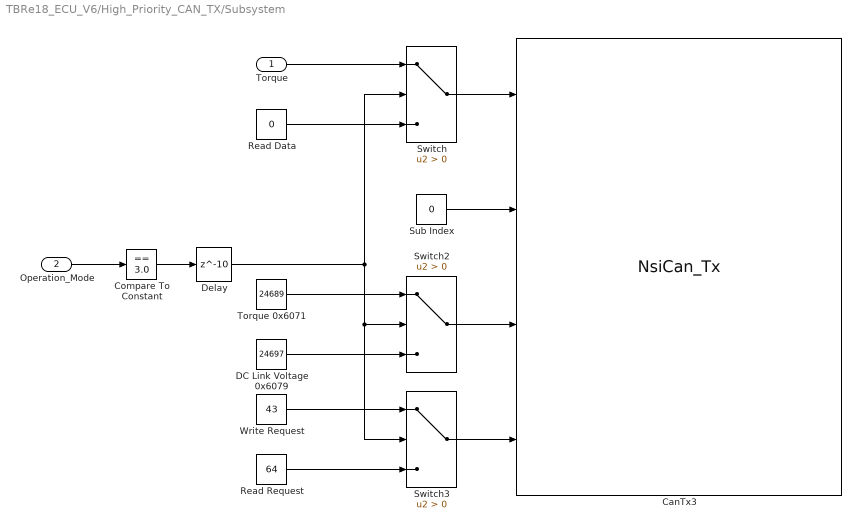
== system TBRe18_ECU_V6/High_Priority_CAN_TX/Subsystem ==
  Torque : Inport
  Operation_Mode : Inport  Port=2
  " Sub Index" : Constant  Value=0  OutDataTypeStr=uint8
  CanTx3 : S-Function  FunctionName=NsiCan_Tx  Parameters=data_can,channel,msg_name,ident,ident_type,dlc,signals  SFunctionDeploymentMode=off  EnableBusSupport=off  mask(MUXlink Can Tx){data_can=1;HIGH_SPEED;500Kbps;120 Ohm;C:\Users\William\Documents\ECU\DBC\TBRe18_DBC_V1.dbc;0;1;HIGH_SPEED;500Kbps;120 Ohm;C:\Users\William\Documents\ECU\DBC\TBRe18_DBC_V1.dbc;0;0;HIGH_SPEED;500Kbps;120 Ohm;C:\Users\l\Desktop\FYP\ECU\DBC\TBRe_DBC_V2.dbc;0;0;HIGH_SPEED;500Kbps;120 Ohm;D:\TOOLS\MUXLINK\R2011b\MUXlink\misc\j1939_adapt.dbc;0;0;HIGH_SPEED;1000Kbps;No;D:\TOOLS\MUXLINK\R2011b\MUXlink\misc\BASE_CAN_MUXLAB4.dbc;0, channel=1, msg_name=MCU_SDO_Request, ident=0x601, ident_type=STD, dlc=8, signals=SDO_Data;1;32;32;MCU_OD_Sub_Index;1;24;8;MCU_OD_Index;1;8;16;SDO_Specifier;1;0;8}
      mask prompts: data_can "data can"; msg_name "msg name"
      mask help: Transmit a frame on a CAN Channel.
      mask init:
      | NsiCan_Tx_InitializationFcn();
      settings: OpenFcn=NsiCan_Tx_OpenFcn();
      mask Help:
      | eval('block=get_param(gcb, ''RTWdata'');')
      | web([docroot '\toolbox\MUXlink\html\blocks/' block.MUXlink_BlockType '.html'])
      mask Callback data_can: NsiCan_Tx_ApplyFcn(1);
      mask Callback channel: NsiCan_Tx_ApplyFcn(2);
      mask Callback msg_name: NsiCan_Tx_ApplyFcn(3);
      mask Callback ident: NsiCan_Tx_ApplyFcn(4);
      mask Callback ident_type: NsiCan_Tx_ApplyFcn(5);
      mask Callback dlc: NsiCan_Tx_ApplyFcn(6);
      mask Callback signals: NsiCan_Tx_ApplyFcn(7);
      mask Display: image(imread('nsi.bmp'));text(0.5, 0.3, 'TX_MCU_SDO_Request_CAN1', 'horizontalAlignment', 'center', 'verticalAlignment', 'base');plot([0.05 0.05 0.05 0.05 0.05 0.05 0.05 0.05 0.05 0.05]); port_label('input',1, 'SDO_Data'); port_label('input',2, 'MCU_OD_Sub_Index'); port_label('input',3, 'MCU_OD_Index'); port_label('input',4, 'SDO_Specifier');
  Compare To Constant : simulink/Logic and Bit Operations/Compare To Constant  relop===  const=3.0  OutDataTypeStr=boolean
  DC Link Voltage 0x6079 : Constant  Value=24697
  Delay : Delay  DelayLength=10  InitialCondition=0
  Read Data : Constant  Value=0
  Read Request : Constant  Value=64
  Switch : Switch  Criteria=u2 > Threshold  OutDataTypeStr=uint32
  Switch2 : Switch  Criteria=u2 > Threshold  OutDataTypeStr=uint16
  Switch3 : Switch  Criteria=u2 > Threshold  OutDataTypeStr=uint8
  Torque 0x6071 : Constant  Value=24689
  Write Request : Constant  Value=43
  wires:
  Switch/1 -> CanTx3/1
  " Sub Index"/1 -> CanTx3/2
  Switch3/1 -> CanTx3/4
  Switch2/1 -> CanTx3/3
  Read Request/1 -> Switch3/3
  Torque/1 -> Switch/1
  Write Request/1 -> Switch3/1
  Delay/1 -> Switch/2, Switch3/2, Switch2/2
  Read Data/1 -> Switch/3
  Torque 0x6071/1 -> Switch2/1
  DC Link Voltage 0x6079/1 -> Switch2/3
  Operation_Mode/1 -> Compare To Constant/1
  Compare To Constant/1 -> Delay/1

== system TBRe18_ECU_V6/Low_Priority_CAN_RX/Init ==

== system TBRe18_ECU_V6/Low_Priority_CAN_TX/BMS_Diagnostics_Data ==
  In1 : Inport

== system TBRe18_ECU_V6/Low_Priority_CAN_TX/CSB_Data ==
  In1 : Inport
